simulink model "NavFilterTestHarness"  (Simulink 7.9)
settings: Solver=FixedStepDiscrete  StartTime=0.0  StopTime=max(IMUtime)  FixedStep=0.001  RelTol=1e-3
undefined symbols (not defined in the file or in its folder): ADSframe, ATTframe, CourseDeg, dAngX, dAngY, dAngZ, dVelX, dVelY, dVelZ, GndSpd, GPSframe, Hgt, IMUframe, IMUtime, LatDeg, LngDeg, MagBiasX, MagBiasY, MagBiasZ, MAGframe, MagX, MagY, MagZ, Pitch, Roll, Veas, VelD, Yaw
libraries: simulink x12
(part 1 of 3)
settings Model: Creator=user  LastModifiedBy=user  SimulationMode=rapid-accelerator
settings DebuggingCC: ParameterPrecisionLossMsg=none
settings SFSimCC: SimParseCustomCode=off

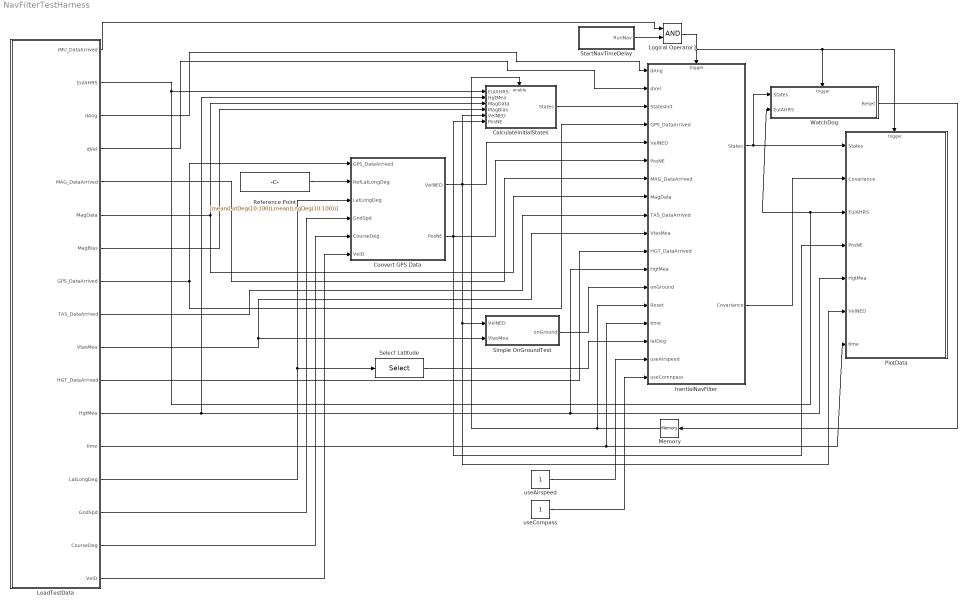
== system NavFilterTestHarness ==
  CalculateInitialStates : Subsystem  TreatAsAtomicUnit=on
  Convert GPS Data : MATLAB Function  TreatAsAtomicUnit=on
  InertialNavFilter : Subsystem
  LoadTestData : Subsystem  TreatAsAtomicUnit=on
  Logical Operator1 : Logic  AllPortsSameDT=off  OutDataTypeStr=boolean
  Memory : Memory  InheritSampleTime=on
  PlotData : Subsystem
  Reference Point : Constant  Value=[mean(LatDeg(10:100)),mean(LngDeg(10:100))]  OutDataTypeStr=single
  Select Latitude : Selector  InputPortWidth=2  IndexOptions=Index vector (dialog)  Indices=1  OutputSizes=1
  Simple OnGroundTest : Subsystem  TreatAsAtomicUnit=on
  StartNavTimeDelay : Subsystem  TreatAsAtomicUnit=on  mask{navStartTime=30}
      mask prompts: navStartTime "Nav Start Time"
  WatchDog : Subsystem  TreatAsAtomicUnit=on
  useAirspeed : Constant  OutDataTypeStr=boolean
  useCompass : Constant  OutDataTypeStr=boolean
  wires:
  LoadTestData/1(IMU_DataArrived) -> Logical Operator1/1
  InertialNavFilter/1(States) -> PlotData/1(States), WatchDog/1(States)
  Logical Operator1/1 -> InertialNavFilter/Trigger, PlotData/Trigger, WatchDog/Trigger
  StartNavTimeDelay/1(RunNav) -> Logical Operator1/2
  InertialNavFilter/2(Covariance) -> PlotData/2(Covariance)
  WatchDog/1(Reset) -> Memory/1
  Memory/1 -> InertialNavFilter/14(Reset), CalculateInitialStates/Enable
  CalculateInitialStates/1(States) -> InertialNavFilter/3(StatesInit)
  Convert GPS Data/2(PosNE) -> InertialNavFilter/6(PosNE), CalculateInitialStates/6(PosNE), PlotData/4(PosNE)
  Convert GPS Data/1(VelNED) -> InertialNavFilter/5(VelNED), CalculateInitialStates/5(VelNED), Simple OnGroundTest/1(VelNED), PlotData/6(VelNED)
  LoadTestData/12(HgtMea) -> CalculateInitialStates/2(HgtMea), PlotData/5(HgtMea), InertialNavFilter/12(HgtMea)
  LoadTestData/6(MagData) -> CalculateInitialStates/3(MagData), InertialNavFilter/8(MagData)
  LoadTestData/7(MagBias) -> CalculateInitialStates/4(MagBias)
  LoadTestData/2(EulAHRS) -> CalculateInitialStates/1(EulAHRS), PlotData/3(EulAHRS), WatchDog/2(EulAHRS)
  LoadTestData/3(dAng) -> InertialNavFilter/1(dAng)
  LoadTestData/4(dVel) -> InertialNavFilter/2(dVel)
  LoadTestData/5(MAG_DataArrived) -> InertialNavFilter/7(MAG_DataArrived)
  LoadTestData/9(TAS_DataArrived) -> InertialNavFilter/9(TAS_DataArrived)
  LoadTestData/10(VtasMea) -> InertialNavFilter/10(VtasMea), Simple OnGroundTest/2(VtasMea)
  LoadTestData/11(HGT_DataArrived) -> InertialNavFilter/11(HGT_DataArrived)
  LoadTestData/13(time) -> InertialNavFilter/15(time), PlotData/7(time)
  Reference Point/1 -> Convert GPS Data/2(RefLatLongDeg)
  LoadTestData/8(GPS_DataArrived) -> Convert GPS Data/1(GPS_DataArrived), InertialNavFilter/4(GPS_DataArrived)
  LoadTestData/14(LatLongDeg) -> Convert GPS Data/3(LatLongDeg), Select Latitude/1
  LoadTestData/15(GndSpd) -> Convert GPS Data/4(GndSpd)
  LoadTestData/16(CourseDeg) -> Convert GPS Data/5(CourseDeg)
  LoadTestData/17(VelD) -> Convert GPS Data/6(VelD)
  Simple OnGroundTest/1(onGround) -> InertialNavFilter/13(onGround)
  Select Latitude/1 -> InertialNavFilter/16(latDeg)
  useAirspeed/1 -> InertialNavFilter/17(useAirspeed)
  useCompass/1 -> InertialNavFilter/18(useComnpass)

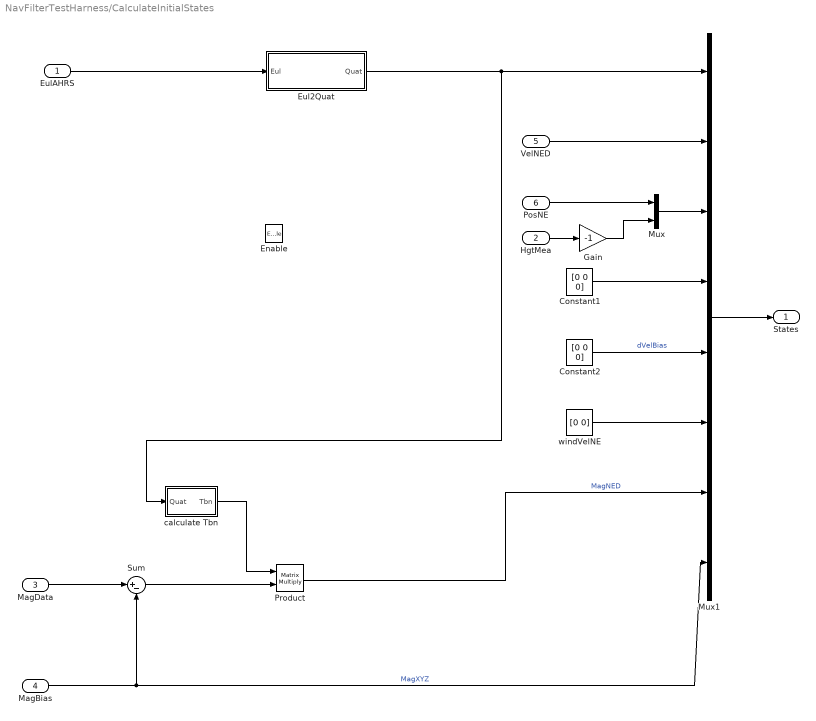
== system NavFilterTestHarness/CalculateInitialStates ==
  EulAHRS : Inport
  HgtMea : Inport  Port=2
  MagData : Inport  Port=3
  MagBias : Inport  Port=4
  VelNED : Inport  Port=5  OutDataTypeStr=single
  PosNE : Inport  Port=6
  Enable : EnablePort
  Constant1 : Constant  Value=[0 0 0]  OutDataTypeStr=single
  Constant2 : Constant  Value=[0 0 0]  OutDataTypeStr=single
  Eul2Quat : Subsystem
  Gain : Gain  Gain=-1
  Mux : Mux  Inputs=2
  Mux1 : Mux  Inputs=8
  Product : Product  Multiplication=Matrix(*)  RndMeth=Zero
  Sum : Sum  Inputs=|+-
  calculate Tbn : Subsystem
  windVelNE : Constant  Value=[0 0]  OutDataTypeStr=single
  States : Outport
  wires:
  Sum/1 -> Product/2
  MagData/1 -> Sum/1
  Eul2Quat/1(Quat) -> Mux1/1, calculate Tbn/1(Quat)
  Mux1/1 -> States/1
  MagBias/1 -> Sum/2, Mux1/8  "MagXYZ"
  windVelNE/1 -> Mux1/6
  Constant2/1 -> Mux1/5  "dVelBias"
  VelNED/1 -> Mux1/2
  Product/1 -> Mux1/7  "MagNED"
  calculate Tbn/1(Tbn) -> Product/1
  EulAHRS/1 -> Eul2Quat/1(Eul)
  Gain/1 -> Mux/2
  PosNE/1 -> Mux/1
  Mux/1 -> Mux1/3
  Constant1/1 -> Mux1/4
  HgtMea/1 -> Gain/1

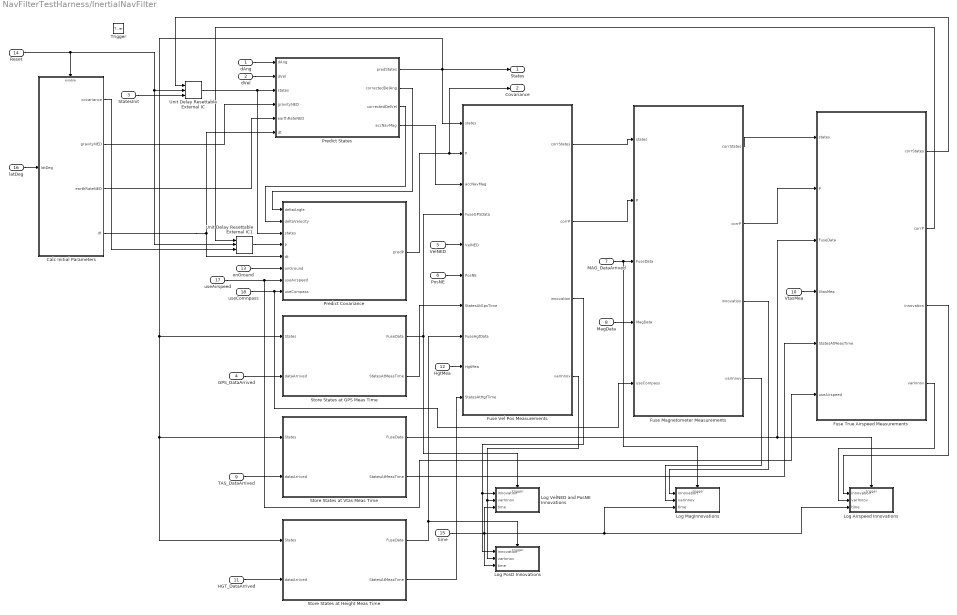
== system NavFilterTestHarness/InertialNavFilter ==
  dAng : Inport  OutDataTypeStr=single  PortDimensions=3
  dVel : Inport  Port=2  OutDataTypeStr=single  PortDimensions=3
  StatesInit : Inport  Port=3  OutDataTypeStr=single  PortDimensions=24
  GPS_DataArrived : Inport  Port=4  OutDataTypeStr=boolean  PortDimensions=1
  VelNED : Inport  Port=5  OutDataTypeStr=single  PortDimensions=3
  PosNE : Inport  Port=6  OutDataTypeStr=single  PortDimensions=2
  MAG_DataArrived : Inport  Port=7  OutDataTypeStr=boolean  PortDimensions=1
  MagData : Inport  Port=8  OutDataTypeStr=single  PortDimensions=3
  TAS_DataArrived : Inport  Port=9  OutDataTypeStr=boolean  PortDimensions=1
  VtasMea : Inport  Port=10  OutDataTypeStr=single  PortDimensions=1
  HGT_DataArrived : Inport  Port=11  OutDataTypeStr=boolean  PortDimensions=1
  HgtMea : Inport  Port=12  OutDataTypeStr=single  PortDimensions=1
  onGround : Inport  Port=13  OutDataTypeStr=boolean  PortDimensions=1
  Reset : Inport  Port=14  OutDataTypeStr=boolean  PortDimensions=1
  time : Inport  Port=15  OutDataTypeStr=double  PortDimensions=1
  latDeg : Inport  Port=16  OutDataTypeStr=single  PortDimensions=1
  useAirspeed : Inport  Port=17  OutDataTypeStr=boolean  PortDimensions=1
  useComnpass : Inport  Port=18  OutDataTypeStr=boolean  PortDimensions=1
  Trigger : TriggerPort  PortDimensions=1
  Calc Initial Parameters : Subsystem
  Fuse Magnetometer Measurements : MATLAB Function  TreatAsAtomicUnit=on
  Fuse True Airspeed Measurements : MATLAB Function  TreatAsAtomicUnit=on
  Fuse Vel Pos Measurements : MATLAB Function  TreatAsAtomicUnit=on
  Log Airspeed Innovations : Subsystem
  Log MagInnovations : Subsystem
  Log PosD Innovations : Subsystem
  Log VelNED and PosNE Innovations : Subsystem
  Predict Covariance : MATLAB Function  TreatAsAtomicUnit=on
  Predict States : MATLAB Function  TreatAsAtomicUnit=on
  Store States at GPS Meas Time : MATLAB Function  TreatAsAtomicUnit=on
  Store States at Height Meas Time : MATLAB Function  TreatAsAtomicUnit=on
  Store States at Vtas Meas Time : MATLAB Function  TreatAsAtomicUnit=on
  Unit Delay Resettable External IC : simulink/Additional Math & Discrete/Additional Discrete/Unit Delay Resettable External IC  tsamp=-1
  Unit Delay Resettable External IC1 : simulink/Additional Math & Discrete/Additional Discrete/Unit Delay Resettable External IC  tsamp=-1
  States : Outport  OutDataTypeStr=single  PortDimensions=24
  Covariance : Outport  Port=2  OutDataTypeStr=single  PortDimensions=[24,24]
  wires:
  StatesInit/1 -> Unit Delay Resettable External IC/3
  Unit Delay Resettable External IC/1 -> Predict Covariance/3(states), Predict States/3(states)
  Predict States/1(predStates) -> States/1, Store States at GPS Meas Time/1(States), Store States at Vtas Meas Time/1(States), Store States at Height Meas Time/1(States), Fuse Vel Pos Measurements/1(states)
  dAng/1 -> Predict States/1(dAng)
  dVel/1 -> Predict States/2(dVel)
  Calc Initial Parameters/2(gravityNED) -> Predict States/4(gravityNED)
  Calc Initial Parameters/4(dt) -> Predict Covariance/5(dt), Predict States/6(dt)
  Calc Initial Parameters/3(earthRateNED) -> Predict States/5(earthRateNED)
  Unit Delay Resettable External IC1/1 -> Predict Covariance/4(P)
  Calc Initial Parameters/1(covariance) -> Unit Delay Resettable External IC1/3
  Predict States/2(correctedDelAng) -> Predict Covariance/1(deltaAngle)
  Predict States/3(correctedDelVel) -> Predict Covariance/2(deltaVelocity)
  GPS_DataArrived/1 -> Store States at GPS Meas Time/2(dataArrived)
  MagData/1 -> Fuse Magnetometer Measurements/4(MagData)
  Fuse Vel Pos Measurements/2(corrP) -> Fuse Magnetometer Measurements/2(P)
  Fuse Vel Pos Measurements/1(corrStates) -> Fuse Magnetometer Measurements/1(states)
  VtasMea/1 -> Fuse True Airspeed Measurements/4(VtasMea)
  Fuse True Airspeed Measurements/2(corrP) -> Unit Delay Resettable External IC1/1
  Fuse True Airspeed Measurements/1(corrStates) -> Unit Delay Resettable External IC/1
  Fuse Vel Pos Measurements/3(innovation) -> Log VelNED and PosNE Innovations/1(innovation), Log PosD Innovations/1(innovation)
  Store States at GPS Meas Time/1(FuseData) -> Log VelNED and PosNE Innovations/Trigger, Fuse Vel Pos Measurements/4(FuseGPSData)
  TAS_DataArrived/1 -> Store States at Vtas Meas Time/2(dataArrived)
  Store States at Vtas Meas Time/1(FuseData) -> Fuse True Airspeed Measurements/3(FuseData), Log Airspeed Innovations/Trigger
  Store States at Vtas Meas Time/2(StatesAtMeasTime) -> Fuse True Airspeed Measurements/5(StatesAtMeasTime)
  Fuse True Airspeed Measurements/3(innovation) -> Log Airspeed Innovations/1(innovation)
  Store States at GPS Meas Time/2(StatesAtMeasTime) -> Fuse Vel Pos Measurements/7(StatesAtGpsTime)
  PosNE/1 -> Fuse Vel Pos Measurements/6(PosNE)
  VelNED/1 -> Fuse Vel Pos Measurements/5(VelNED)
  Fuse Vel Pos Measurements/4(varInnov) -> Log VelNED and PosNE Innovations/2(varInnov), Log PosD Innovations/2(varInnov)
  Fuse True Airspeed Measurements/4(varInnov) -> Log Airspeed Innovations/2(varInnov)
  HGT_DataArrived/1 -> Store States at Height Meas Time/2(dataArrived)
  Store States at Height Meas Time/1(FuseData) -> Fuse Vel Pos Measurements/8(FuseHgtData), Log PosD Innovations/Trigger
  Store States at Height Meas Time/2(StatesAtMeasTime) -> Fuse Vel Pos Measurements/10(StatesAtHgtTime)
  HgtMea/1 -> Fuse Vel Pos Measurements/9(HgtMea)
  MAG_DataArrived/1 -> Fuse Magnetometer Measurements/3(FuseData), Log MagInnovations/Trigger
  Fuse Magnetometer Measurements/3(innovation) -> Log MagInnovations/1(innovation)
  Fuse Magnetometer Measurements/4(varInnov) -> Log MagInnovations/2(varInnov)
  Fuse Magnetometer Measurements/1(corrStates) -> Fuse True Airspeed Measurements/1(states)
  Fuse Magnetometer Measurements/2(corrP) -> Fuse True Airspeed Measurements/2(P)
  time/1 -> Log VelNED and PosNE Innovations/3(time), Log MagInnovations/3(time), Log Airspeed Innovations/3(time), Log PosD Innovations/3(time)
  Predict Covariance/1(predP) -> Covariance/1, Fuse Vel Pos Measurements/2(P)
  Predict States/4(accNavMag) -> Fuse Vel Pos Measurements/3(accNavMag)
  Reset/1 -> Unit Delay Resettable External IC/2, Unit Delay Resettable External IC1/2, Calc Initial Parameters/Enable
  onGround/1 -> Predict Covariance/6(onGround)
  latDeg/1 -> Calc Initial Parameters/1(latDeg)
  useComnpass/1 -> Predict Covariance/8(useCompass), Fuse Magnetometer Measurements/5(useCompass)
  useAirspeed/1 -> Predict Covariance/7(useAirspeed), Fuse True Airspeed Measurements/6(useAirspeed)

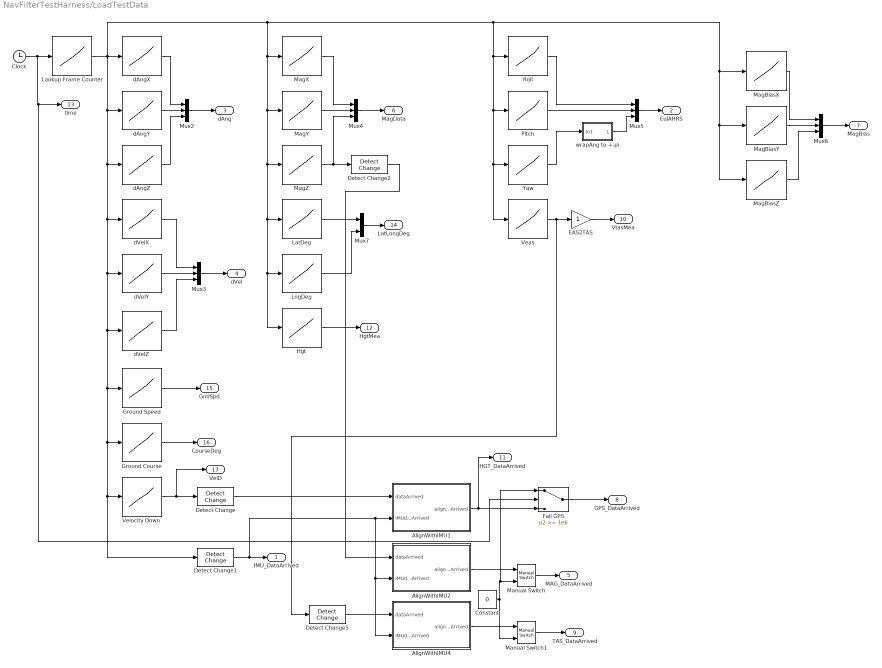
== system NavFilterTestHarness/LoadTestData ==
  AlignWithIMU1 : Subsystem
  AlignWithIMU2 : Subsystem
  AlignWithIMU4 : Subsystem
  Clock : Clock
  Constant : Constant  Value=0  OutDataTypeStr=boolean
  Detect Change{,1..2,5} (4 alike) : simulink/Logic and Bit Operations/Detect Change  vinit=0  InputProcessing=Inherited  OutDataTypeStr=boolean
  EAS2TAS : Gain
  Fail GPS : Switch  Threshold=1e6
  Ground Course : Lookup_n-D  NumberOfTableDimensions=1  BreakpointsForDimension1=GPSframe  BeginIndexSearchUsingPreviousIndexResult=on  Table=CourseDeg  InterpMethod=Flat  OutDataTypeStr=single  RndMeth=Simplest  InputSameDT=on
  Ground Speed : Lookup_n-D  NumberOfTableDimensions=1  BreakpointsForDimension1=GPSframe  BeginIndexSearchUsingPreviousIndexResult=on  Table=GndSpd  InterpMethod=Flat  OutDataTypeStr=single  RndMeth=Simplest  InputSameDT=on
  Hgt : Lookup_n-D  NumberOfTableDimensions=1  BreakpointsForDimension1=GPSframe  BeginIndexSearchUsingPreviousIndexResult=on  Table=Hgt  InterpMethod=Flat  OutDataTypeStr=single  RndMeth=Simplest  InputSameDT=on
  LatDeg : Lookup_n-D  NumberOfTableDimensions=1  BreakpointsForDimension1=GPSframe  BeginIndexSearchUsingPreviousIndexResult=on  Table=LatDeg  InterpMethod=Flat  OutDataTypeStr=single  RndMeth=Simplest  InputSameDT=on
  LngDeg : Lookup_n-D  NumberOfTableDimensions=1  BreakpointsForDimension1=GPSframe  BeginIndexSearchUsingPreviousIndexResult=on  Table=LngDeg  InterpMethod=Flat  OutDataTypeStr=single  RndMeth=Simplest  InputSameDT=on
  Lookup Frame Counter : Lookup_n-D  NumberOfTableDimensions=1  BreakpointsForDimension1=IMUtime  BeginIndexSearchUsingPreviousIndexResult=on  Table=IMUframe  InterpMethod=Flat  DiagnosticForOutOfRangeInput=Error  RndMeth=Simplest  InputSameDT=on
  MagBiasX : Lookup_n-D  NumberOfTableDimensions=1  BreakpointsForDimension1=MAGframe  BeginIndexSearchUsingPreviousIndexResult=on  Table=MagBiasX  InterpMethod=Flat  OutDataTypeStr=single  RndMeth=Simplest  InputSameDT=on
  MagBiasY : Lookup_n-D  NumberOfTableDimensions=1  BreakpointsForDimension1=MAGframe  BeginIndexSearchUsingPreviousIndexResult=on  Table=MagBiasY  InterpMethod=Flat  OutDataTypeStr=single  RndMeth=Simplest  InputSameDT=on
  MagBiasZ : Lookup_n-D  NumberOfTableDimensions=1  BreakpointsForDimension1=MAGframe  BeginIndexSearchUsingPreviousIndexResult=on  Table=MagBiasZ  InterpMethod=Flat  OutDataTypeStr=single  RndMeth=Simplest  InputSameDT=on
  MagX : Lookup_n-D  NumberOfTableDimensions=1  BreakpointsForDimension1=MAGframe  BeginIndexSearchUsingPreviousIndexResult=on  Table=MagX  InterpMethod=Flat  OutDataTypeStr=single  RndMeth=Simplest  InputSameDT=on
  MagY : Lookup_n-D  NumberOfTableDimensions=1  BreakpointsForDimension1=MAGframe  BeginIndexSearchUsingPreviousIndexResult=on  Table=MagY  InterpMethod=Flat  OutDataTypeStr=single  RndMeth=Simplest  InputSameDT=on
  MagZ : Lookup_n-D  NumberOfTableDimensions=1  BreakpointsForDimension1=MAGframe  BeginIndexSearchUsingPreviousIndexResult=on  Table=MagZ  InterpMethod=Flat  OutDataTypeStr=single  RndMeth=Simplest  InputSameDT=on
  Manual Switch : simulink/Signal Routing/Manual Switch  sw=1  action=0  varsize=off
  Manual Switch1 : simulink/Signal Routing/Manual Switch  sw=1  action=0  varsize=off
  Mux{2..6} (5 alike) : Mux  Inputs=3
  Mux7 : Mux  Inputs=2
  Pitch : Lookup_n-D  NumberOfTableDimensions=1  BreakpointsForDimension1=ATTframe  BeginIndexSearchUsingPreviousIndexResult=on  Table=Pitch  InterpMethod=Flat  OutDataTypeStr=single  RndMeth=Simplest  InputSameDT=on
  Roll : Lookup_n-D  NumberOfTableDimensions=1  BreakpointsForDimension1=ATTframe  BeginIndexSearchUsingPreviousIndexResult=on  Table=Roll  InterpMethod=Flat  OutDataTypeStr=single  RndMeth=Simplest  InputSameDT=on
  Veas : Lookup_n-D  NumberOfTableDimensions=1  BreakpointsForDimension1=ADSframe  BeginIndexSearchUsingPreviousIndexResult=on  Table=Veas  InterpMethod=Flat  OutDataTypeStr=single  RndMeth=Simplest  InputSameDT=on
  Velocity Down : Lookup_n-D  NumberOfTableDimensions=1  BreakpointsForDimension1=GPSframe  BeginIndexSearchUsingPreviousIndexResult=on  Table=VelD  InterpMethod=Flat  OutDataTypeStr=single  RndMeth=Simplest  InputSameDT=on
  Yaw : Lookup_n-D  NumberOfTableDimensions=1  BreakpointsForDimension1=ATTframe  BeginIndexSearchUsingPreviousIndexResult=on  Table=Yaw  InterpMethod=Flat  OutDataTypeStr=single  RndMeth=Simplest  InputSameDT=on
  dAngX : Lookup_n-D  NumberOfTableDimensions=1  BreakpointsForDimension1=IMUframe  BeginIndexSearchUsingPreviousIndexResult=on  Table=dAngX  InterpMethod=Flat  DiagnosticForOutOfRangeInput=Error  OutDataTypeStr=single  RndMeth=Simplest  InputSameDT=on
  dAngY : Lookup_n-D  NumberOfTableDimensions=1  BreakpointsForDimension1=IMUframe  BeginIndexSearchUsingPreviousIndexResult=on  Table=dAngY  InterpMethod=Flat  DiagnosticForOutOfRangeInput=Error  OutDataTypeStr=single  RndMeth=Simplest  InputSameDT=on
  dAngZ : Lookup_n-D  NumberOfTableDimensions=1  BreakpointsForDimension1=IMUframe  BeginIndexSearchUsingPreviousIndexResult=on  Table=dAngZ  InterpMethod=Flat  DiagnosticForOutOfRangeInput=Error  OutDataTypeStr=single  RndMeth=Simplest  InputSameDT=on
  dVelX : Lookup_n-D  NumberOfTableDimensions=1  BreakpointsForDimension1=IMUframe  BeginIndexSearchUsingPreviousIndexResult=on  Table=dVelX  InterpMethod=Flat  DiagnosticForOutOfRangeInput=Error  OutDataTypeStr=single  RndMeth=Simplest  InputSameDT=on
  dVelY : Lookup_n-D  NumberOfTableDimensions=1  BreakpointsForDimension1=IMUframe  BeginIndexSearchUsingPreviousIndexResult=on  Table=dVelY  InterpMethod=Flat  DiagnosticForOutOfRangeInput=Error  OutDataTypeStr=single  RndMeth=Simplest  InputSameDT=on
  dVelZ : Lookup_n-D  NumberOfTableDimensions=1  BreakpointsForDimension1=IMUframe  BeginIndexSearchUsingPreviousIndexResult=on  Table=dVelZ  InterpMethod=Flat  DiagnosticForOutOfRangeInput=Error  OutDataTypeStr=single  RndMeth=Simplest  InputSameDT=on
  wrapAng to +-pi : Subsystem
  IMU_DataArrived : Outport  OutDataTypeStr=boolean
  EulAHRS : Outport  Port=2  OutDataTypeStr=single
  dAng : Outport  Port=3  OutDataTypeStr=single
  dVel : Outport  Port=4  OutDataTypeStr=single
  MAG_DataArrived : Outport  Port=5  OutDataTypeStr=boolean
  MagData : Outport  Port=6  OutDataTypeStr=single
  MagBias : Outport  Port=7  OutDataTypeStr=single
  GPS_DataArrived : Outport  Port=8  OutDataTypeStr=boolean
  TAS_DataArrived : Outport  Port=9  OutDataTypeStr=boolean
  VtasMea : Outport  Port=10  OutDataTypeStr=single
  HGT_DataArrived : Outport  Port=11  OutDataTypeStr=boolean
  HgtMea : Outport  Port=12  OutDataTypeStr=single
  time : Outport  Port=13  OutDataTypeStr=double
  LatLongDeg : Outport  Port=14  OutDataTypeStr=single
  GndSpd : Outport  Port=15  OutDataTypeStr=single
  CourseDeg : Outport  Port=16  OutDataTypeStr=single
  VelD : Outport  Port=17  OutDataTypeStr=single
  wires:
  Lookup Frame Counter/1 -> dAngX/1, dAngY/1, dAngZ/1, dVelX/1, dVelY/1, dVelZ/1, Ground Speed/1, Ground Course/1, Velocity Down/1, Detect Change1/1, MagX/1, MagY/1, MagZ/1, LatDeg/1, Hgt/1, LngDeg/1, Roll/1, Pitch/1, Yaw/1, Veas/1, MagBiasX/1, MagBiasZ/1, MagBiasY/1
  Velocity Down/1 -> Detect Change/1, VelD/1
  Mux2/1 -> dAng/1
  dAngX/1 -> Mux2/1
  dAngY/1 -> Mux2/2
  dAngZ/1 -> Mux2/3
  Mux3/1 -> dVel/1
  dVelY/1 -> Mux3/2
  dVelX/1 -> Mux3/1
  dVelZ/1 -> Mux3/3
  Mux4/1 -> MagData/1
  MagY/1 -> Mux4/2
  MagX/1 -> Mux4/1
  MagZ/1 -> Mux4/3, Detect Change2/1
  Roll/1 -> Mux5/1
  Pitch/1 -> Mux5/2
  Yaw/1 -> wrapAng to +-pi/1(In1)
  Mux5/1 -> EulAHRS/1
  wrapAng to +-pi/1(Out1) -> Mux5/3
  Detect Change/1 -> AlignWithIMU1/1(dataArrived)
  Detect Change1/1 -> IMU_DataArrived/1, AlignWithIMU1/2(IMUdataArrived), AlignWithIMU2/2(IMUdataArrived), AlignWithIMU4/2(IMUdataArrived)
  Veas/1 -> Detect Change5/1, EAS2TAS/1
  AlignWithIMU1/1(alignedDataArrived) -> HGT_DataArrived/1, Fail GPS/3
  Detect Change2/1 -> AlignWithIMU2/1(dataArrived)
  AlignWithIMU2/1(alignedDataArrived) -> Manual Switch/1
  Manual Switch/1 -> MAG_DataArrived/1
  Constant/1 -> Fail GPS/1, Manual Switch/2, Manual Switch1/2
  Detect Change5/1 -> AlignWithIMU4/1(dataArrived)
  EAS2TAS/1 -> VtasMea/1
  Manual Switch1/1 -> TAS_DataArrived/1
  AlignWithIMU4/1(alignedDataArrived) -> Manual Switch1/1
  Mux6/1 -> MagBias/1
  MagBiasY/1 -> Mux6/2
  MagBiasX/1 -> Mux6/1
  MagBiasZ/1 -> Mux6/3
  Fail GPS/1 -> GPS_DataArrived/1
  Clock/1 -> Lookup Frame Counter/1, Fail GPS/2, time/1
  Hgt/1 -> HgtMea/1
  LatDeg/1 -> Mux7/1
  LngDeg/1 -> Mux7/2
  Mux7/1 -> LatLongDeg/1
  Ground Speed/1 -> GndSpd/1
  Ground Course/1 -> CourseDeg/1

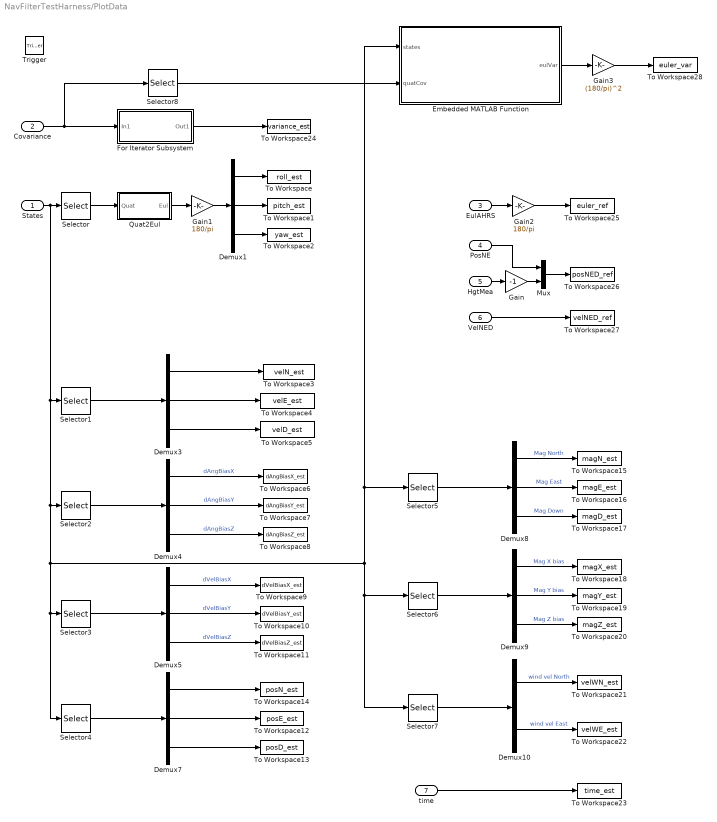
== system NavFilterTestHarness/PlotData ==
  States : Inport
  Covariance : Inport  Port=2  PortDimensions=[24,24]
  EulAHRS : Inport  Port=3
  PosNE : Inport  Port=4
  HgtMea : Inport  Port=5
  VelNED : Inport  Port=6
  time : Inport  Port=7  OutDataTypeStr=double  PortDimensions=1
  Trigger : TriggerPort  PortDimensions=1
  Demux{1,3..5,7..9} (7 alike) : Demux  Outputs=3
  Demux10 : Demux  Outputs=2
  Embedded MATLAB Function : MATLAB Function  TreatAsAtomicUnit=on
  For Iterator Subsystem : Subsystem  TreatAsAtomicUnit=on
  Gain : Gain  Gain=-1
  Gain1 : Gain  Gain=180/pi
  Gain2 : Gain  Gain=180/pi
  Gain3 : Gain  Gain=(180/pi)^2
  Mux : Mux  Inputs=2
  Quat2Eul : Subsystem
  Selector : Selector  InputPortWidth=24  IndexOptions=Index vector (dialog)  Indices=[1:4]  OutputSizes=1
  Selector1 : Selector  InputPortWidth=24  IndexOptions=Index vector (dialog)  Indices=[5:7]  OutputSizes=1
  Selector2 : Selector  InputPortWidth=24  IndexOptions=Index vector (dialog)  Indices=[11:13]  OutputSizes=1
  Selector3 : Selector  InputPortWidth=24  IndexOptions=Index vector (dialog)  Indices=[14:16]  OutputSizes=1
  Selector4 : Selector  InputPortWidth=24  IndexOptions=Index vector (dialog)  Indices=[8:10]  OutputSizes=1
  Selector5 : Selector  InputPortWidth=24  IndexOptions=Index vector (dialog)  Indices=[19:21]  OutputSizes=1
  Selector6 : Selector  InputPortWidth=24  IndexOptions=Index vector (dialog)  Indices=[22:24]  OutputSizes=1
  Selector7 : Selector  InputPortWidth=24  IndexOptions=Index vector (dialog)  Indices=[17:18]  OutputSizes=1
  Selector8 : Selector  NumberOfDimensions=2  InputPortWidth=3  IndexOptions=Index vector (dialog),Index vector (dialog)  Indices=[1:4],[1:4]  OutputSizes=1,1
  To Workspace : ToWorkspace  VariableName=roll_est  SampleTime=-1
  To Workspace1 : ToWorkspace  VariableName=pitch_est  SampleTime=-1
  To Workspace10 : ToWorkspace  VariableName=dVelBiasY_est  SampleTime=-1
  To Workspace11 : ToWorkspace  VariableName=dVelBiasZ_est  SampleTime=-1
  To Workspace12 : ToWorkspace  VariableName=posE_est  SampleTime=-1
  To Workspace13 : ToWorkspace  VariableName=posD_est  SampleTime=-1
  To Workspace14 : ToWorkspace  VariableName=posN_est  SampleTime=-1
  To Workspace15 : ToWorkspace  VariableName=magN_est  SampleTime=-1
  To Workspace16 : ToWorkspace  VariableName=magE_est  SampleTime=-1
  To Workspace17 : ToWorkspace  VariableName=magD_est  SampleTime=-1
  To Workspace18 : ToWorkspace  VariableName=magX_est  SampleTime=-1
  To Workspace19 : ToWorkspace  VariableName=magY_est  SampleTime=-1
  To Workspace2 : ToWorkspace  VariableName=yaw_est  SampleTime=-1
  To Workspace20 : ToWorkspace  VariableName=magZ_est  SampleTime=-1
  To Workspace21 : ToWorkspace  VariableName=velWN_est  SampleTime=-1
  To Workspace22 : ToWorkspace  VariableName=velWE_est  SampleTime=-1
  To Workspace23 : ToWorkspace  VariableName=time_est  SampleTime=-1
  To Workspace24 : ToWorkspace  VariableName=variance_est  SampleTime=-1
  To Workspace25 : ToWorkspace  VariableName=euler_ref  SampleTime=-1
  To Workspace26 : ToWorkspace  VariableName=posNED_ref  SampleTime=-1
  To Workspace27 : ToWorkspace  VariableName=velNED_ref  SampleTime=-1
  To Workspace28 : ToWorkspace  VariableName=euler_var  SampleTime=-1
  To Workspace3 : ToWorkspace  VariableName=velN_est  SampleTime=-1
  To Workspace4 : ToWorkspace  VariableName=velE_est  SampleTime=-1
  To Workspace5 : ToWorkspace  VariableName=velD_est  SampleTime=-1
  To Workspace6 : ToWorkspace  VariableName=dAngBiasX_est  SampleTime=-1
  To Workspace7 : ToWorkspace  VariableName=dAngBiasY_est  SampleTime=-1
  To Workspace8 : ToWorkspace  VariableName=dAngBiasZ_est  SampleTime=-1
  To Workspace9 : ToWorkspace  VariableName=dVelBiasX_est  SampleTime=-1
  wires:
  Quat2Eul/1(Eul) -> Gain1/1
  Selector/1 -> Quat2Eul/1(Quat)
  States/1 -> Selector2/1, Selector4/1, Selector3/1, Embedded MATLAB Function/1(states), Selector5/1, Selector6/1, Selector7/1, Selector1/1, Selector/1
  Gain1/1 -> Demux1/1
  Selector1/1 -> Demux3/1
  Selector2/1 -> Demux4/1
  Selector3/1 -> Demux5/1
  Demux4/1 -> To Workspace6/1  "dAngBiasX"
  Selector4/1 -> Demux7/1
  Selector5/1 -> Demux8/1
  Selector6/1 -> Demux9/1
  Selector7/1 -> Demux10/1
  Demux4/3 -> To Workspace8/1  "dAngBiasZ"
  Demux4/2 -> To Workspace7/1  "dAngBiasY"
  Demux5/1 -> To Workspace9/1  "dVelBiasX"
  Demux5/2 -> To Workspace10/1  "dVelBiasY"
  Demux5/3 -> To Workspace11/1  "dVelBiasZ"
  Demux8/1 -> To Workspace15/1  "Mag North"
  Demux8/2 -> To Workspace16/1  "Mag East"
  Demux8/3 -> To Workspace17/1  "Mag Down"
  Demux9/1 -> To Workspace18/1  "Mag X bias"
  Demux9/2 -> To Workspace19/1  "Mag Y bias"
  Demux9/3 -> To Workspace20/1  "Mag Z bias"
  Demux10/1 -> To Workspace21/1  "wind vel North"
  Demux10/2 -> To Workspace22/1  "wind vel East"
  time/1 -> To Workspace23/1
  Demux7/1 -> To Workspace14/1
  Demux7/2 -> To Workspace12/1
  Demux7/3 -> To Workspace13/1
  Demux3/1 -> To Workspace3/1
  Demux3/2 -> To Workspace4/1
  Demux3/3 -> To Workspace5/1
  Demux1/3 -> To Workspace2/1
  Demux1/2 -> To Workspace1/1
  Demux1/1 -> To Workspace/1
  Covariance/1 -> Selector8/1, For Iterator Subsystem/1(In1)
  EulAHRS/1 -> Gain2/1
  HgtMea/1 -> Gain/1
  PosNE/1 -> Mux/1
  Mux/1 -> To Workspace26/1
  VelNED/1 -> To Workspace27/1
  Gain/1 -> Mux/2
  Gain2/1 -> To Workspace25/1
  Embedded MATLAB Function/1(eulVar) -> Gain3/1
  For Iterator Subsystem/1(Out1) -> To Workspace24/1
  Selector8/1 -> Embedded MATLAB Function/2(quatCov)
  Gain3/1 -> To Workspace28/1

== system NavFilterTestHarness/Simple OnGroundTest ==
  VelNED : Inport
  VtasMea : Inport  Port=2
  Logical Operator : Logic  AllPortsSameDT=off  OutDataTypeStr=boolean
  Test Airspeed : simulink/Logic and Bit Operations/Compare To Constant  relop=<  const=8  OutDataTypeStr=boolean
  Test Ground Spee : simulink/Logic and Bit Operations/Compare To Constant  relop=<  const=2  OutDataTypeStr=boolean
  gndSpd : Fcn  Expr=sqrt(u(1)^2 + u(2)^2)
  onGround : Outport
  wires:
  gndSpd/1 -> Test Ground Spee/1
  Test Airspeed/1 -> Logical Operator/2
  Test Ground Spee/1 -> Logical Operator/1
  VelNED/1 -> gndSpd/1
  VtasMea/1 -> Test Airspeed/1
  Logical Operator/1 -> onGround/1

== system NavFilterTestHarness/StartNavTimeDelay ==
  Clock : Clock
  Compare To Constant2 : simulink/Logic and Bit Operations/Compare To Constant  relop=>  const=navStartTime  OutDataTypeStr=boolean
  RunNav : Outport
  wires:
  Clock/1 -> Compare To Constant2/1
  Compare To Constant2/1 -> RunNav/1

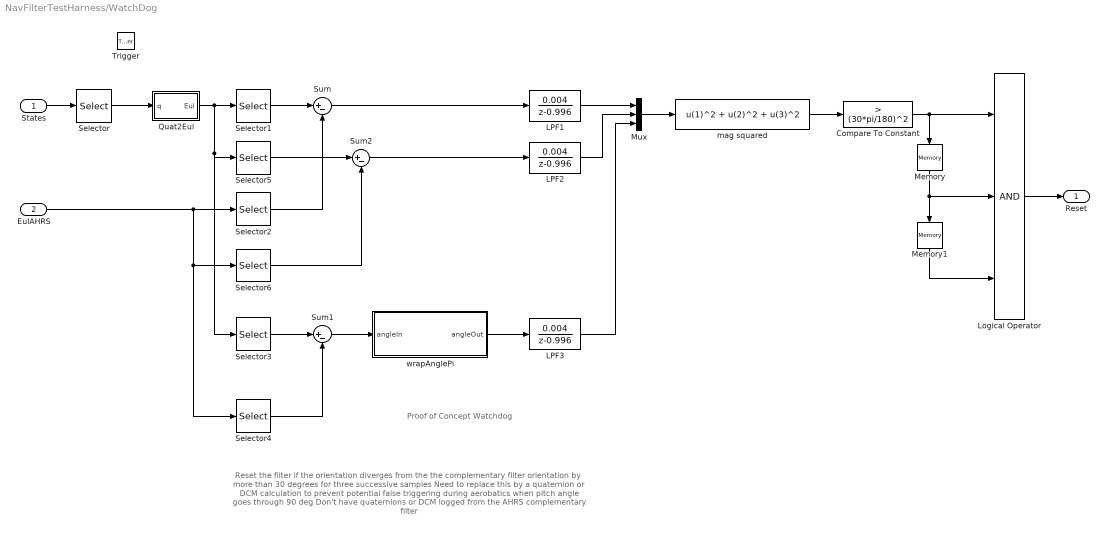
== system NavFilterTestHarness/WatchDog ==
  note: Reset the filter if the orientation diverges from the the complementary filter orientation  by more than 30 degrees for three successive samples
      | Need to replace this by a quaternion or DCM calculation to prevent potential false triggering during aerobatics when pitch angle goes through 90 deg
      | Don't have quaternions or DCM logged from the AHRS complementary filter
  note: Proof of Concept Watchdog
  States : Inport
  EulAHRS : Inport  Port=2
  Trigger : TriggerPort  PortDimensions=1
  Compare To Constant : simulink/Logic and Bit Operations/Compare To Constant  relop=>  const=(30*pi/180)^2  OutDataTypeStr=boolean
  LPF1 : DiscreteTransferFcn  Numerator=0.004  Denominator=[1 -0.996]
  LPF2 : DiscreteTransferFcn  Numerator=0.004  Denominator=[1 -0.996]
  LPF3 : DiscreteTransferFcn  Numerator=0.004  Denominator=[1 -0.996]
  Logical Operator : Logic  Inputs=3  AllPortsSameDT=off  OutDataTypeStr=boolean
  Memory : Memory  InheritSampleTime=on
  Memory1 : Memory  InheritSampleTime=on
  Mux : Mux  Inputs=3
  Quat2Eul : Subsystem
  Selector : Selector  InputPortWidth=24  IndexOptions=Index vector (dialog)  Indices=[1:4]  OutputSizes=1
  Selector1 : Selector  InputPortWidth=3  IndexOptions=Index vector (dialog)  Indices=1  OutputSizes=1
  Selector2 : Selector  InputPortWidth=3  IndexOptions=Index vector (dialog)  Indices=1  OutputSizes=1
  Selector3 : Selector  InputPortWidth=3  IndexOptions=Index vector (dialog)  Indices=3  OutputSizes=1
  Selector4 : Selector  InputPortWidth=3  IndexOptions=Index vector (dialog)  Indices=3  OutputSizes=1
  Selector5 : Selector  InputPortWidth=3  IndexOptions=Index vector (dialog)  Indices=2  OutputSizes=1
  Selector6 : Selector  InputPortWidth=3  IndexOptions=Index vector (dialog)  Indices=2  OutputSizes=1
  Sum : Sum  Inputs=|+-
  Sum1 : Sum  Inputs=|+-
  Sum2 : Sum  Inputs=|+-
  mag squared : Fcn  Expr=u(1)^2 + u(2)^2 + u(3)^2
  wrapAnglePi : MATLAB Function  TreatAsAtomicUnit=on
  Reset : Outport  OutDataTypeStr=boolean  PortDimensions=1
  wires:
  Selector/1 -> Quat2Eul/1(q)
  States/1 -> Selector/1
  Quat2Eul/1(Eul) -> Selector1/1, Selector3/1, Selector5/1
  EulAHRS/1 -> Selector2/1, Selector4/1, Selector6/1
  Selector3/1 -> Sum1/1
  Selector4/1 -> Sum1/2
  Sum1/1 -> wrapAnglePi/1(angleIn)
  Sum/1 -> LPF1/1
  wrapAnglePi/1(angleOut) -> LPF3/1
  Mux/1 -> mag squared/1
  mag squared/1 -> Compare To Constant/1
  Compare To Constant/1 -> Logical Operator/1, Memory/1
  Logical Operator/1 -> Reset/1
  Memory/1 -> Logical Operator/2, Memory1/1
  Memory1/1 -> Logical Operator/3
  Selector1/1 -> Sum/1
  Selector2/1 -> Sum/2
  Selector5/1 -> Sum2/1
  Selector6/1 -> Sum2/2
  Sum2/1 -> LPF2/1
  LPF1/1 -> Mux/1
  LPF2/1 -> Mux/2
  LPF3/1 -> Mux/3

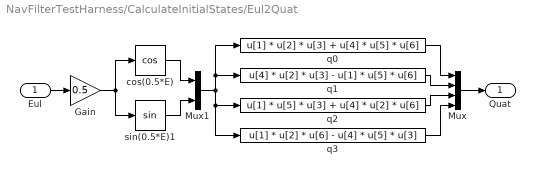
== system NavFilterTestHarness/CalculateInitialStates/Eul2Quat ==
  Eul : Inport
  Gain : Gain  Gain=0.5  SaturateOnIntegerOverflow=on  OutDataTypeStr=Inherit: Same as input  ParamDataTypeStr=Inherit: Same as input
  Mux : Mux
  Mux1 : Mux  Inputs=[3 3]
  cos(0.5*E) : Trigonometry  Operator=cos
  q0 : Fcn  Expr=u[1] * u[2] * u[3] + u[4] * u[5] * u[6]
  q1 : Fcn  Expr=u[4] * u[2] * u[3] - u[1] * u[5] * u[6]
  q2 : Fcn  Expr=u[1] * u[5] * u[3] + u[4] * u[2] * u[6]
  q3 : Fcn  Expr=u[1] * u[2] * u[6] - u[4] * u[5] * u[3]
  sin(0.5*E)1 : Trigonometry
  Quat : Outport
  wires:
  Eul/1 -> Gain/1
  Gain/1 -> cos(0.5*E)/1, sin(0.5*E)1/1
  cos(0.5*E)/1 -> Mux1/1
  sin(0.5*E)1/1 -> Mux1/2
  q0/1 -> Mux/1
  Mux/1 -> Quat/1
  q1/1 -> Mux/2
  q2/1 -> Mux/3
  q3/1 -> Mux/4
  Mux1/1 -> q0/1, q1/1, q3/1, q2/1

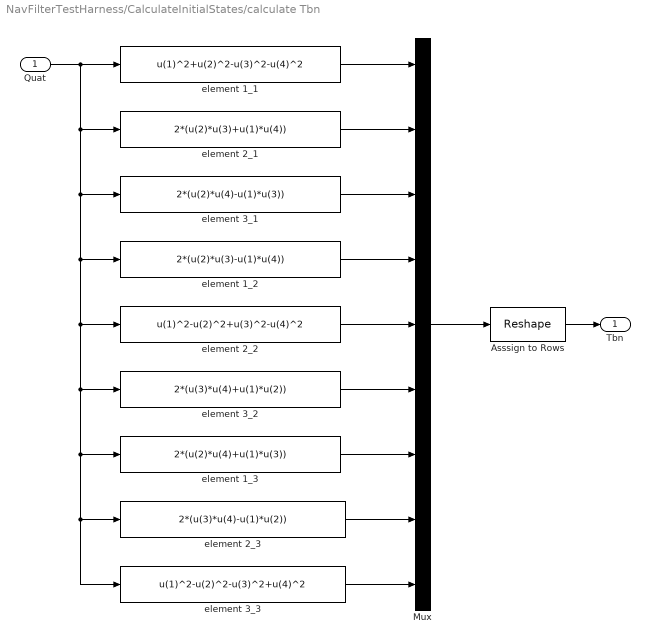
== system NavFilterTestHarness/CalculateInitialStates/calculate Tbn ==
  Quat : Inport  PortDimensions=4
  Asssign to Rows : Reshape  OutputDimensionality=Customize  OutputDimensions=[3,3]
  Mux : Mux  Inputs=9
  element 1_1 : Fcn  Expr=u(1)^2+u(2)^2-u(3)^2-u(4)^2
  element 1_2 : Fcn  Expr=2*(u(2)*u(3)-u(1)*u(4))
  element 1_3 : Fcn  Expr=2*(u(2)*u(4)+u(1)*u(3))
  element 2_1 : Fcn  Expr=2*(u(2)*u(3)+u(1)*u(4))
  element 2_2 : Fcn  Expr=u(1)^2-u(2)^2+u(3)^2-u(4)^2
  element 2_3 : Fcn  Expr=2*(u(3)*u(4)-u(1)*u(2))
  element 3_1 : Fcn  Expr=2*(u(2)*u(4)-u(1)*u(3))
  element 3_2 : Fcn  Expr=2*(u(3)*u(4)+u(1)*u(2))
  element 3_3 : Fcn  Expr=u(1)^2-u(2)^2-u(3)^2+u(4)^2
  Tbn : Outport
  wires:
  Mux/1 -> Asssign to Rows/1
  element 1_1/1 -> Mux/1
  element 2_1/1 -> Mux/2
  element 3_1/1 -> Mux/3
  element 1_2/1 -> Mux/4
  element 2_2/1 -> Mux/5
  element 3_2/1 -> Mux/6
  element 1_3/1 -> Mux/7
  element 2_3/1 -> Mux/8
  element 3_3/1 -> Mux/9
  Asssign to Rows/1 -> Tbn/1
  Quat/1 -> element 1_1/1, element 3_3/1, element 2_3/1, element 1_3/1, element 3_2/1, element 2_2/1, element 1_2/1, element 3_1/1, element 2_1/1

== system NavFilterTestHarness/InertialNavFilter/Calc Initial Parameters ==
  latDeg : Inport  OutDataTypeStr=single  PortDimensions=1
  Enable : EnablePort  PropagateVarSize=During execution
  Embedded MATLAB Function : MATLAB Function  TreatAsAtomicUnit=on
  covariance : Outport
  gravityNED : Outport  Port=2  PortDimensions=3
  earthRateNED : Outport  Port=3  PortDimensions=3
  dt : Outport  Port=4  PortDimensions=1  InitialOutput=0
  wires:
  Embedded MATLAB Function/1(covariance) -> covariance/1
  Embedded MATLAB Function/2(gravityNED) -> gravityNED/1
  Embedded MATLAB Function/3(earthRateNED) -> earthRateNED/1
  latDeg/1 -> Embedded MATLAB Function/1(latDeg)
  Embedded MATLAB Function/4(dt) -> dt/1

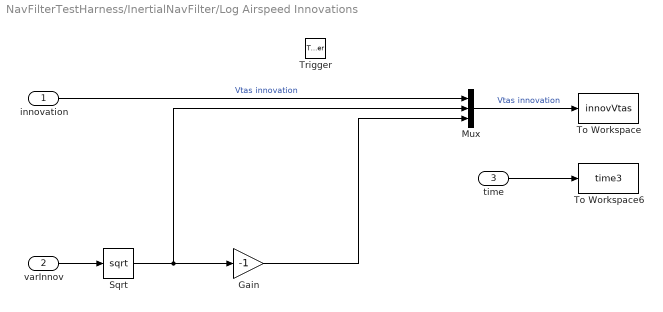
== system NavFilterTestHarness/InertialNavFilter/Log Airspeed Innovations ==
  innovation : Inport
  varInnov : Inport  Port=2
  time : Inport  Port=3
  Trigger : TriggerPort  PortDimensions=1
  Gain : Gain  Gain=-1
  Mux : Mux  Inputs=3
  Sqrt : Sqrt  SaturateOnIntegerOverflow=on
  To Workspace : ToWorkspace  VariableName=innovVtas  SampleTime=-1
  To Workspace6 : ToWorkspace  VariableName=time3  SampleTime=-1
  wires:
  Mux/1 -> To Workspace/1  "Vtas innovation"
  innovation/1 -> Mux/1  "Vtas innovation"
  varInnov/1 -> Sqrt/1
  Sqrt/1 -> Mux/2, Gain/1
  Gain/1 -> Mux/3
  time/1 -> To Workspace6/1

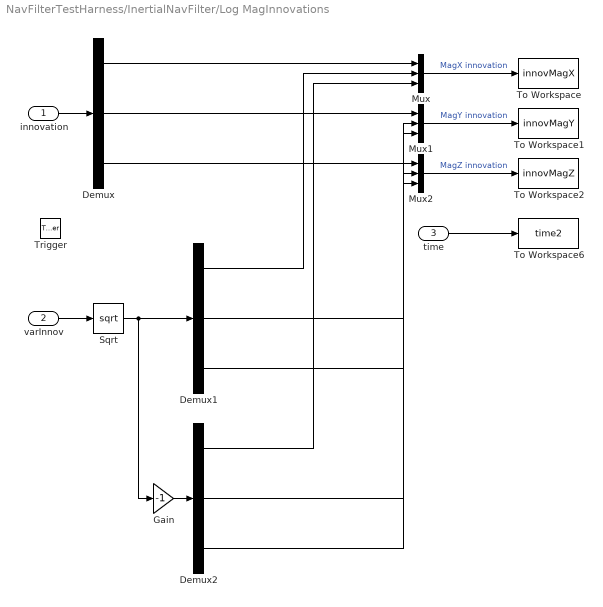
== system NavFilterTestHarness/InertialNavFilter/Log MagInnovations ==
  innovation : Inport
  varInnov : Inport  Port=2
  time : Inport  Port=3
  Trigger : TriggerPort  PortDimensions=1
  Demux : Demux  Outputs=3
  Demux1 : Demux  Outputs=3
  Demux2 : Demux  Outputs=3
  Gain : Gain  Gain=-1
  Mux : Mux  Inputs=3
  Mux1 : Mux  Inputs=3
  Mux2 : Mux  Inputs=3
  Sqrt : Sqrt  SaturateOnIntegerOverflow=on
  To Workspace : ToWorkspace  VariableName=innovMagX  SampleTime=-1
  To Workspace1 : ToWorkspace  VariableName=innovMagY  SampleTime=-1
  To Workspace2 : ToWorkspace  VariableName=innovMagZ  SampleTime=-1
  To Workspace6 : ToWorkspace  VariableName=time2  SampleTime=-1
  wires:
  Mux2/1 -> To Workspace2/1  "MagZ innovation"
  Mux1/1 -> To Workspace1/1  "MagY innovation"
  Mux/1 -> To Workspace/1  "MagX innovation"
  Demux2/3 -> Mux2/3
  Demux1/3 -> Mux2/2
  Demux/3 -> Mux2/1
  Demux2/2 -> Mux1/3
  Demux1/2 -> Mux1/2
  Demux/2 -> Mux1/1
  Demux2/1 -> Mux/3
  Demux1/1 -> Mux/2
  Demux/1 -> Mux/1
  Gain/1 -> Demux2/1
  Sqrt/1 -> Gain/1, Demux1/1
  varInnov/1 -> Sqrt/1
  innovation/1 -> Demux/1
  time/1 -> To Workspace6/1

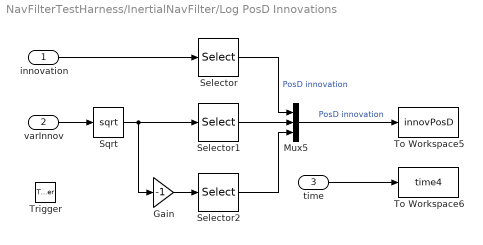
== system NavFilterTestHarness/InertialNavFilter/Log PosD Innovations ==
  innovation : Inport
  varInnov : Inport  Port=2
  time : Inport  Port=3
  Trigger : TriggerPort  PortDimensions=1
  Gain : Gain  Gain=-1
  Mux5 : Mux  Inputs=3
  Selector : Selector  InputPortWidth=6  IndexOptions=Index vector (dialog)  Indices=6  OutputSizes=1
  Selector1 : Selector  InputPortWidth=6  IndexOptions=Index vector (dialog)  Indices=6  OutputSizes=1
  Selector2 : Selector  InputPortWidth=6  IndexOptions=Index vector (dialog)  Indices=6  OutputSizes=1
  Sqrt : Sqrt  SaturateOnIntegerOverflow=on
  To Workspace5 : ToWorkspace  VariableName=innovPosD  SampleTime=-1
  To Workspace6 : ToWorkspace  VariableName=time4  SampleTime=-1
  wires:
  time/1 -> To Workspace6/1
  Mux5/1 -> To Workspace5/1  "PosD innovation"
  Selector1/1 -> Mux5/2
  Selector/1 -> Mux5/1  "PosD innovation"
  Gain/1 -> Selector2/1
  Sqrt/1 -> Gain/1, Selector1/1
  varInnov/1 -> Sqrt/1
  innovation/1 -> Selector/1
  Selector2/1 -> Mux5/3

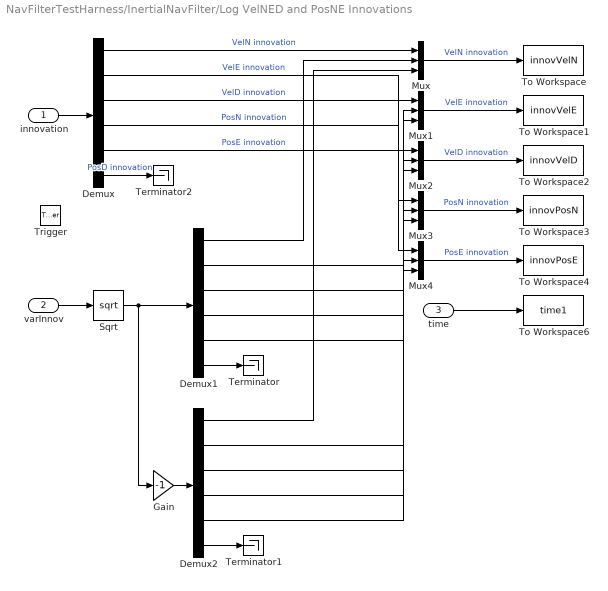
== system NavFilterTestHarness/InertialNavFilter/Log VelNED and PosNE Innovations ==
  innovation : Inport
  varInnov : Inport  Port=2
  time : Inport  Port=3
  Trigger : TriggerPort  PortDimensions=1
  Demux : Demux  Outputs=6
  Demux1 : Demux  Outputs=6
  Demux2 : Demux  Outputs=6
  Gain : Gain  Gain=-1
  Mux{,1..4} (5 alike) : Mux  Inputs=3
  Sqrt : Sqrt  SaturateOnIntegerOverflow=on
  Terminator : Terminator
  Terminator1 : Terminator
  Terminator2 : Terminator
  To Workspace : ToWorkspace  VariableName=innovVelN  SampleTime=-1
  To Workspace1 : ToWorkspace  VariableName=innovVelE  SampleTime=-1
  To Workspace2 : ToWorkspace  VariableName=innovVelD  SampleTime=-1
  To Workspace3 : ToWorkspace  VariableName=innovPosN  SampleTime=-1
  To Workspace4 : ToWorkspace  VariableName=innovPosE  SampleTime=-1
  To Workspace6 : ToWorkspace  VariableName=time1  SampleTime=-1
  wires:
  innovation/1 -> Demux/1
  varInnov/1 -> Sqrt/1
  Sqrt/1 -> Demux1/1, Gain/1
  Gain/1 -> Demux2/1
  Demux/1 -> Mux/1  "VelN innovation"
  Demux1/1 -> Mux/2
  Demux2/1 -> Mux/3
  Demux/2 -> Mux1/1  "VelE innovation"
  Demux1/2 -> Mux1/2
  Demux2/2 -> Mux1/3
  Demux/3 -> Mux2/1  "VelD innovation"
  Demux1/3 -> Mux2/2
  Demux2/3 -> Mux2/3
  Demux/4 -> Mux3/1  "PosN innovation"
  Demux1/4 -> Mux3/2
  Demux2/4 -> Mux3/3
  Demux/5 -> Mux4/1  "PosE innovation"
  Demux1/5 -> Mux4/2
  Demux2/5 -> Mux4/3
  Mux/1 -> To Workspace/1  "VelN innovation"
  Mux1/1 -> To Workspace1/1  "VelE innovation"
  Mux2/1 -> To Workspace2/1  "VelD innovation"
  Mux3/1 -> To Workspace3/1  "PosN innovation"
  Mux4/1 -> To Workspace4/1  "PosE innovation"
  time/1 -> To Workspace6/1
  Demux1/6 -> Terminator/1
  Demux2/6 -> Terminator1/1
  Demux/6 -> Terminator2/1  "PosD innovation"

== system NavFilterTestHarness/LoadTestData/AlignWithIMU1 ==
  dataArrived : Inport
  IMUdataArrived : Inport  Port=2
  Logical Operator : Logic  Operator=OR  AllPortsSameDT=off  OutDataTypeStr=boolean
  Logical Operator1 : Logic  AllPortsSameDT=off  OutDataTypeStr=boolean
  Logical Operator2 : Logic  Operator=NOT  AllPortsSameDT=off  OutDataTypeStr=boolean
  Memory : Memory
  alignedDataArrived : Outport
  wires:
  Logical Operator/1 -> Logical Operator1/1, alignedDataArrived/1
  Memory/1 -> Logical Operator/2
  Logical Operator1/1 -> Memory/1
  Logical Operator2/1 -> Logical Operator1/2
  dataArrived/1 -> Logical Operator/1
  IMUdataArrived/1 -> Logical Operator2/1

== system NavFilterTestHarness/LoadTestData/AlignWithIMU2 ==
  dataArrived : Inport
  IMUdataArrived : Inport  Port=2
  Logical Operator : Logic  Operator=OR  AllPortsSameDT=off  OutDataTypeStr=boolean
  Logical Operator1 : Logic  AllPortsSameDT=off  OutDataTypeStr=boolean
  Logical Operator2 : Logic  Operator=NOT  AllPortsSameDT=off  OutDataTypeStr=boolean
  Memory : Memory
  alignedDataArrived : Outport
  wires:
  Logical Operator/1 -> Logical Operator1/1, alignedDataArrived/1
  Memory/1 -> Logical Operator/2
  Logical Operator1/1 -> Memory/1
  Logical Operator2/1 -> Logical Operator1/2
  dataArrived/1 -> Logical Operator/1
  IMUdataArrived/1 -> Logical Operator2/1

== system NavFilterTestHarness/LoadTestData/AlignWithIMU4 ==
  dataArrived : Inport
  IMUdataArrived : Inport  Port=2
  Logical Operator : Logic  Operator=OR  AllPortsSameDT=off  OutDataTypeStr=boolean
  Logical Operator1 : Logic  AllPortsSameDT=off  OutDataTypeStr=boolean
  Logical Operator2 : Logic  Operator=NOT  AllPortsSameDT=off  OutDataTypeStr=boolean
  Memory : Memory
  alignedDataArrived : Outport
  wires:
  IMUdataArrived/1 -> Logical Operator2/1
  dataArrived/1 -> Logical Operator/1
  Logical Operator2/1 -> Logical Operator1/2
  Logical Operator1/1 -> Memory/1
  Memory/1 -> Logical Operator/2
  Logical Operator/1 -> alignedDataArrived/1, Logical Operator1/1

== system NavFilterTestHarness/LoadTestData/wrapAng to +-pi ==
  In1 : Inport  OutDataTypeStr=single
  If : If  IfExpression=u1 > single(pi)
  If Action Subsystem : Subsystem  TreatAsAtomicUnit=on
  If Action Subsystem1 : Subsystem  TreatAsAtomicUnit=on
  Merge : Merge
  Out1 : Outport  OutDataTypeStr=single
  wires:
  In1/1 -> If Action Subsystem1/1(In1), If Action Subsystem/1(In1), If/1
  If/2 -> If Action Subsystem/Action
  If/1 -> If Action Subsystem1/Action
  If Action Subsystem/1(Out1) -> Merge/1
  If Action Subsystem1/1(Out1) -> Merge/2
  Merge/1 -> Out1/1

== system NavFilterTestHarness/PlotData/For Iterator Subsystem ==
  In1 : Inport
  Assignment : Assignment  OutputInitialize=Specify size for each dimension in table  IndexOptions=Index vector (port)  Indices=1  OutputSizes=24
  For Iterator : ForIterator  IterationLimit=24
  Select5 : Selector  NumberOfDimensions=2  InputPortWidth=3  IndexOptions=Index vector (port),Index vector (port)  Indices=1,1  OutputSizes=1,1
  Out1 : Outport
  wires:
  In1/1 -> Select5/1
  For Iterator/1 -> Select5/2, Select5/3, Assignment/2
  Select5/1 -> Assignment/1
  Assignment/1 -> Out1/1

== system NavFilterTestHarness/PlotData/Quat2Eul ==
  Quat : Inport  PortDimensions=4
  Mux : Mux  Inputs=3
  Pitch : Fcn  Expr=-asin(2*(u[2]*u[4]-u[1]*u[3]))
  Roll : Fcn  Expr=atan2(2*(u[3]*u[4]+u[1]*u[2] ) , u[1]^2-u[2]^2-u[3]^2+u[4]^2)
  Yaw : Fcn  Expr=atan2(2*(u[2]*u[3]+u[1]*u[4] ) , u[1]^2+u[2]^2-u[3]^2-u[4]^2)
  Eul : Outport
  wires:
  Mux/1 -> Eul/1
  Roll/1 -> Mux/1
  Pitch/1 -> Mux/2
  Quat/1 -> Roll/1, Pitch/1, Yaw/1
  Yaw/1 -> Mux/3

== system NavFilterTestHarness/WatchDog/Quat2Eul ==
  q : Inport  PortDimensions=4
  Mux : Mux  Inputs=3
  phi : Fcn  Expr=atan2(2*(u[3]*u[4]+u[1]*u[2] ) , u[1]^2-u[2]^2-u[3]^2+u[4]^2)
  psi : Fcn  Expr=atan2(2*(u[2]*u[3]+u[1]*u[4] ) , u[1]^2+u[2]^2-u[3]^2-u[4]^2)
  theta : Fcn  Expr=-asin(2*(u[2]*u[4]-u[1]*u[3]))
  Eul : Outport
  wires:
  Mux/1 -> Eul/1
  phi/1 -> Mux/1
  theta/1 -> Mux/2
  q/1 -> phi/1, theta/1, psi/1
  psi/1 -> Mux/3

== system NavFilterTestHarness/LoadTestData/wrapAng to +-pi/If Action Subsystem ==
  In1 : Inport
  Action Port : ActionPort  ActionType=else
  Out1 : Outport
  wires:
  In1/1 -> Out1/1

== system NavFilterTestHarness/LoadTestData/wrapAng to +-pi/If Action Subsystem1 ==
  In1 : Inport
  Action Port : ActionPort  ActionType=then
  Add : Sum  Inputs=+-
  Constant : Constant  Value=2*pi  OutDataTypeStr=single
  Out1 : Outport
  wires:
  In1/1 -> Add/1
  Add/1 -> Out1/1
  Constant/1 -> Add/2

== matlab function WatchDog/wrapAnglePi ==
  data: angleOut output double; angleIn input double
function angleOut   = wrapAnglePi(angleIn)
%#codegen

if abs(angleIn) <= pi
    angleOut = angleIn;
elseif  angleIn < -pi
    angleOut = angleIn + 2*pi;
elseif angleIn > pi
    angleOut = angleIn - 2*pi;
else
    angleOut = angleIn;
end

end

== matlab function InertialNavFilter/Predict States ==
  data: dAng input double; dVel input double; states input double; predStates output double; gravityNED input double; earthRateNED input double; dt input double; correctedDelAng output double; correctedDelVel output double; accNavMag output double
%#codegen
function [predStates,correctedDelAng,correctedDelVel,accNavMag]  = UpdateStrapdownEquationsNED(dAng, ...
    dVel, ...
    states, ...
    gravityNED, ...
    earthRateNED, ...
    dt)

% define persistent variables for previous delta angle and velocity which
% are required for sculling and coning error corrections
persistent prevDelAng;
if isempty(prevDelAng)
    prevDelAng = single([0;0;0]);
end
persistent prevDelVel;
if isempty(prevDelVel)
    prevDelVel = single([0;0;0]);
end
persistent Tbn;
if isempty(Tbn)
    Tbn = single(eye(3));
end

% Remove sensor bias errors
dVel = dVel - states(14:16);
dAng = dAng - states(11:13);

% Apply rotational and skulling corrections
correctedDelVel= dVel + ...
    0.5*cross(prevDelAng + dAng , prevDelVel + dVel) + 1/6*cross(prevDelAng + dAng , cross(prevDelAng + dAng , prevDelVel + dVel)) + ... % rotational correction
    1/12*(cross(prevDelAng , dVel) + cross(prevDelVel , dAng)); % sculling correction

% Apply corrections for earths rotation rate and coning errors
correctedDelAng   = dAng - transpose(Tbn)*earthRateNED*dt + 1/12*cross(prevDelAng , dAng);

% Save current measurements
prevDelAng = dAng;
prevDelVel = dVel;

% Initialise the updated state vector
predStates   = states;

% Convert the rotation vector to its equivalent quaternion
rotationMag = sqrt(correctedDelAng(1)^2 + correctedDelAng(2)^2 + correctedDelAng(3)^2);
if rotationMag<1e-12
  deltaQuat = single([1;0;0;0]);
else
  deltaQuat = [cos(0.5*rotationMag); correctedDelAng/rotationMag*sin(0.5*rotationMag)];
end

% Update the quaternions by rotating from the previous attitude through
% the delta angle rotation quaternion
qUpdated = [states(1)*deltaQuat(1)-transpose(states(2:4))*deltaQuat(2:4); states(1)*deltaQuat(2:4) + deltaQuat(1)*states(2:4) + cross(states(2:4),deltaQuat(2:4))];

% Normalise the quaternions and update the quaternion states
quatMag = sqrt(qUpdated(1)^2 + qUpdated(2)^2 + qUpdated(3)^2 + qUpdated(4)^2);
if (quatMag < 1e-16)
    predStates(1:4) = qUpdated;
else
    predStates(1:4) = qUpdated / quatMag;
end

% Calculate the body to nav cosine matrix
Tbn = [predStates(1)^2 + predStates(2)^2 - predStates(3)^2 - predStates(4)^2, 2*(predStates(2)*predStates(3) - predStates(1)*predStates(4)), 2*(predStates(2)*predStates(4) + predStates(1)*predStates(3));...
      2*(predStates(2)*predStates(3) + predStates(1)*predStates(4)), predStates(1)^2 - predStates(2)^2 + predStates(3)^2 - predStates(4)^2, 2*(predStates(3)*predStates(4) - predStates(1)*predStates(2));...
      2*(predStates(2)*predStates(4)-predStates(1)*predStates(3)), 2*(predStates(3)*predStates(4) + predStates(1)*predStates(2)), predStates(1)^2 - predStates(2)^2 - predStates(3)^2 + predStates(4)^2];
  
% transform body delta velocities to delta velocities in the nav frame
delVelNav = Tbn * correctedDelVel + gravityNED*dt;

% calculate the magnitude of the nav acceleration (required for GPS
% variance estimation)
accNavMag = sqrt(delVelNav(1)^2 + delVelNav(2)^2 + delVelNav(3)^2) / dt;

% If calculating position save previous velocity
lastVelocity = predStates(5:7);

% Sum delta velocities to get velocity after removing gravitational skew and correcting for transport rate
predStates(5:7) = states(5:7) + delVelNav;


% If calculating postions, do a trapezoidal integration for position
predStates(8:10)     = states(8:10) + 0.5*(predStates(5:7) + lastVelocity)*dt;

% Copy the remaining states across
predStates(11:24) = states(11:24);

end
